simulink model "q2a"  (R2024a)
settings: Solver=VariableStepAuto  StartTime=0.0  StopTime=5  MaxStep=1e-4  RelTol=1e-3
settings Model: Creator=SHINE MOHAN S  LastModifiedBy=SHINE MOHAN S

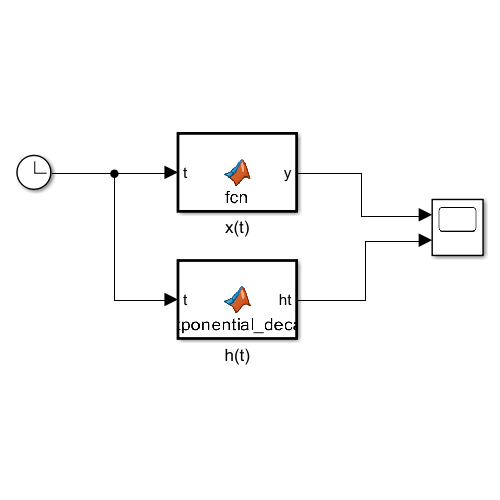
[thumbnail: Simulink's stored preview of the top-level diagram]
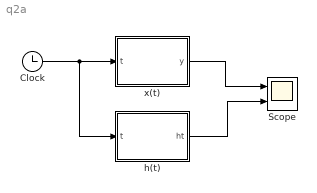
== system q2a ==
  Clock : Clock
  Scope : Scope  NumInputPorts=2
  h(t) : MATLAB Function  TreatAsAtomicUnit=on
  x(t) : MATLAB Function  TreatAsAtomicUnit=on
  wires:
  Clock/1 -> h(t)/1(t), x(t)/1(t)
  x(t)/1(y) -> Scope/1
  h(t)/1(ht) -> Scope/2

== matlab function q2a/x(t) ==
  data: t input; y output
function y = fcn(t)
    if t >= 0 && t < 3
        y = 1;
    else
        y = 0;
    end
end

== matlab function q2a/h(t) ==
  data: t input; ht output
function ht = exponential_decay(t)
    ht = exp(-t);
end
